simulink model "Sim"  (R2019a)
settings: Solver=VariableStepAuto  StartTime=0.0  StopTime=231884  RelTol=1e-3
values from neighbouring files (symbols this model uses):
  f0 = f(1)    [Flywheel.m]
  Fifsd = ku/p    (= 0.2925)    [Flywheel.m]
  J = 2*capacity/(w_max^2)    [Flywheel.m]
  Kp_omega = 2*ksides*J*wn_omega - f1    [Flywheel.m]
  Kpd = 2*ksides*Ld*wn_d - Rs    (= 1.68186666667)    [Flywheel.m]
  Kpq = 2*ksides*Lq*wn_q - Rs    (= 1.70245045045)    [Flywheel.m]
  Ld = 0.00259    [Flywheel.m]
  Lq = 0.00262    [Flywheel.m]
  p = 4    [Flywheel.m]
  Rs = 0.0952    [Flywheel.m]
  Ti_omega = Kp_omega/(J*wn_omega*wn_omega)    [Flywheel.m]
  Tid = Kpd/(Ld*wn_d*wn_d)    (= 0.00270358455882)    [Flywheel.m]
  Tiq = Kpq/(Lq*wn_q*wn_q)    (= 0.00270533684609)    [Flywheel.m]
settings Model: Creator=ayhans  LastModifiedBy=DELL
settings DataIOCC: ReturnWorkspaceOutputs=off
settings DebuggingCC: ArithmeticOperatorsInVariantConditions=warning

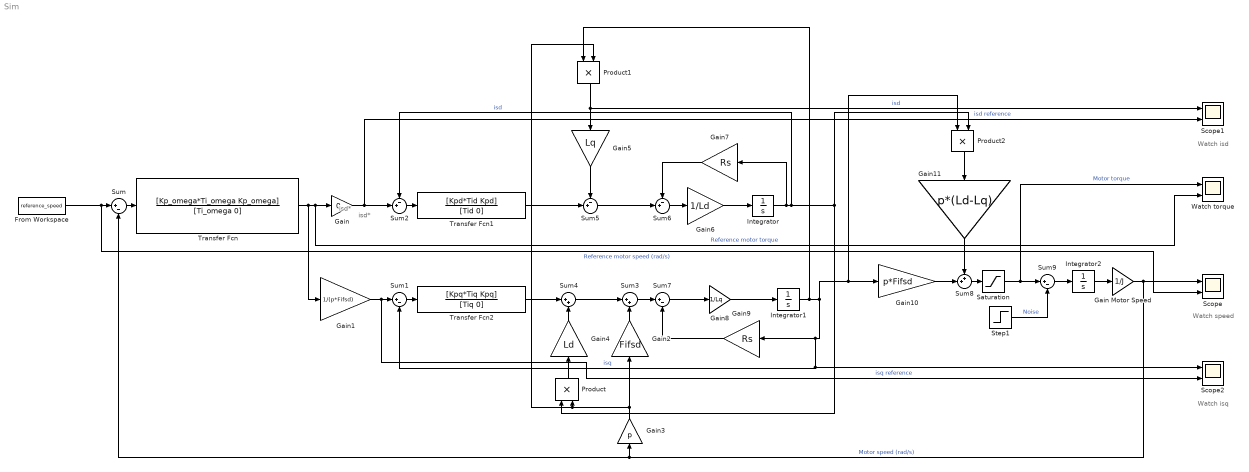
== system Sim ==
  note: Watch isd
  note: Watch speed
  note: Watch isq
  note: isd*
  note: isd*
  From Workspace : FromWorkspace  VariableName=reference_speed  SampleTime=0
  Gain : Gain  Gain=0
  "Gain Motor Speed " : Gain  Gain=1/J
  Gain1 : Gain  Gain=1/(p*Fifsd)
  Gain10 : Gain  Gain=p*Fifsd
  Gain11 : Gain  Gain=p*(Ld-Lq)
  Gain2 : Gain  Gain=Fifsd
  Gain3 : Gain  Gain=p
  Gain4 : Gain  Gain=Ld
  Gain5 : Gain  Gain=Lq
  Gain6 : Gain  Gain=1/Ld
  Gain7 : Gain  Gain=Rs
  Gain8 : Gain  Gain=1/Lq
  Gain9 : Gain  Gain=Rs
  Integrator : Integrator
  Integrator1 : Integrator
  Integrator2 : Integrator
  Product : Product
  Product1 : Product
  Product2 : Product
  Saturation : Saturate  UpperLimit=2500000000000000000  LowerLimit=-2500000000000000000
  Scope : Scope  NumInputPorts=2
  Scope1 : Scope  NumInputPorts=2
  Scope2 : Scope  NumInputPorts=2
  Step1 : Step  Time=25  After=f0  SampleTime=0
  Sum{,1,7,9} (4 alike) : Sum  Inputs=|+-
  Sum2 : Sum  Inputs=-+|
  Sum3 : Sum  Inputs=|++
  Sum4 : Sum  Inputs=|++
  Sum5 : Sum  Inputs=-+|
  Sum6 : Sum  Inputs=-+|
  Sum8 : Sum  Inputs=++|
  Transfer Fcn : TransferFcn  Numerator=[Kp_omega*Ti_omega Kp_omega]  Denominator=[Ti_omega 0]
  Transfer Fcn1 : TransferFcn  Numerator=[Kpd*Tid Kpd]  Denominator=[Tid 0]
  Transfer Fcn2 : TransferFcn  Numerator=[Kpq*Tiq Kpq]  Denominator=[Tiq 0]
  Watch torque : Scope  NumInputPorts=2
  wires:
  From Workspace/1 -> Scope/2, Sum/1  "Reference motor speed (rad/s)"
  Sum/1 -> Transfer Fcn/1
  Transfer Fcn/1 -> Gain1/1, Watch torque/2, Gain/1  "Reference motor torque"
  Gain/1 -> Scope1/2, Sum2/2  "isd reference"
  Sum2/1 -> Transfer Fcn1/1
  Sum1/1 -> Transfer Fcn2/1
  Gain1/1 -> Scope2/2, Sum1/1  "isq reference"
  Sum4/1 -> Sum3/1
  Transfer Fcn1/1 -> Sum5/2
  Transfer Fcn2/1 -> Sum4/1
  "Gain Motor Speed "/1 -> Sum/2, Gain3/1, Scope/1  "Motor speed (rad/s)"
  Gain2/1 -> Sum3/2
  Gain3/1 -> Product1/2, Product/2, Gain2/1
  Gain4/1 -> Sum4/2
  Product/1 -> Gain4/1
  Sum5/1 -> Sum6/2
  Gain5/1 -> Sum5/1
  Product1/1 -> Gain5/1, Scope1/1  "isd"
  Sum6/1 -> Gain6/1
  Gain6/1 -> Integrator/1
  Integrator/1 -> Product/1, Product2/2, Sum2/1, Gain7/1  "isd"
  Gain7/1 -> Sum6/1
  Gain8/1 -> Integrator1/1
  Sum7/1 -> Gain8/1
  Integrator1/1 -> Sum1/2, Scope2/1, Gain9/1, Gain10/1, Product2/1, Product1/1  "isq"
  Sum3/1 -> Sum7/1
  Gain9/1 -> Sum7/2
  Gain10/1 -> Sum8/2
  Product2/1 -> Gain11/1
  Gain11/1 -> Sum8/1
  Integrator2/1 -> "Gain Motor Speed "/1
  Sum9/1 -> Integrator2/1
  Step1/1 -> Sum9/2  "Noise"
  Saturation/1 -> Watch torque/1, Sum9/1  "Motor torque"
  Sum8/1 -> Saturation/1
